simulink model "CBE_145_HW4_P1b"  (R2021b)
settings: Solver=VariableStepAuto  StartTime=0.0  StopTime=100  RelTol=1e-3
settings Model: Creator=Jesus Vergara  LastModifiedBy=brame
settings SolverCC: AlgebraicLoopSolver=TrustRegion
settings DataIOCC: InspectSignalLogs=on  LoggingToFile=on
settings DebuggingCC: SFMachineParentedDataDiag=warning

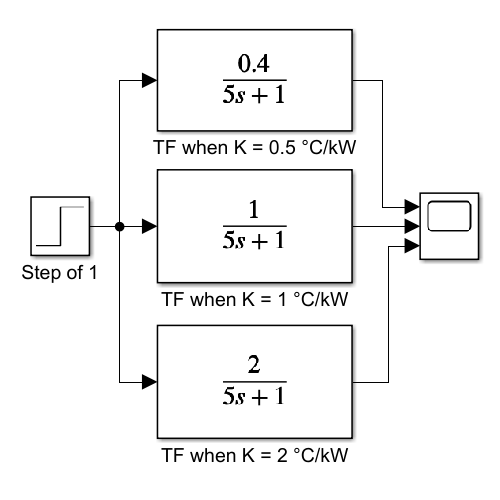
[thumbnail: Simulink's stored preview of the top-level diagram]
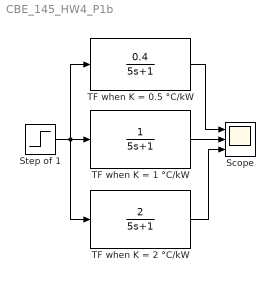
== system CBE_145_HW4_P1b ==
  Scope : Scope  NumInputPorts=3
  Step of 1 : Step  SampleTime=0
  TF when K = 0.5 °C/kW : TransferFcn  Numerator=[0.4]  Denominator=[5 1]
  TF when K = 1 °C/kW : TransferFcn  Denominator=[5 1]
  TF when K = 2 °C/kW : TransferFcn  Numerator=[2]  Denominator=[5 1]
  wires:
  Step of 1/1 -> TF when K = 0.5 °C/kW/1, TF when K = 2 °C/kW/1, TF when K = 1 °C/kW/1
  TF when K = 1 °C/kW/1 -> Scope/2
  TF when K = 0.5 °C/kW/1 -> Scope/1
  TF when K = 2 °C/kW/1 -> Scope/3
